simulink model "RealLifeTrainModel"  (R2024a)
settings: Solver=ode1  StartTime=0.0  StopTime=Inf  FixedStep=0.001  RelTol=1e-3
PostLoadFcn:
  | , if any(exist('dsrtsu_mdlpostloadfcn', 'file') ~= 0), dsrtsu_mdlpostloadfcn('Execute', bdroot); end,
InitFcn:
  | , if any(exist('rtifpga_mdlclblib', 'file') ~= 0), rtifpga_mdlclblib('Init', bdroot); end,
undefined symbols (not defined in the file): DiscIntNeverNeededParam
libraries: deeplib x29, svdutilitieslib x28, simulink x8, eeGeneralControl x8, rti1202lib_adc_class1 x6, rti1202serlib x5, spsEdgeDetectorLib x5, rtiemclib x2, rti1202lib_dac_class1 x1
(part 7 of 8)

== matlab function RealLifeTrainModel/ContractionMetricFilterSystem3/Normalize_Policy ==
  data: u input; y output
function y = fcn(u)

max_Fload =  569.629505294963
min_Fload = -610.339671010468

max_Fhyd = 729.261146885585
min_Fhyd = -777.489547410502

max_DFload = 123011.265014651
min_DFload = -142353.177843906

max_DFhyd = 219994.429294316
min_DFhyd = -270882.694509076

max_Pa = 12037835.3221229
min_Pa = 1849925.22965178

max_Pb = 14831789.6053956
min_Pb = 2808786.27887814

max_x = 0.082368752
min_x = 0.01990812

max_Dx = 0.682789396628826
min_Dx = -0.578996654196926

out = [1,1,1,1,1,1,1,1,1]

out(1) = (u(1) - min_Fhyd)/(max_Fhyd - min_Fhyd);
out(2) = (u(2) - min_DFhyd)/(max_DFhyd - min_DFhyd);
out(3) = (u(3) - min_Fload)/(max_Fload - min_Fload);
out(4) = (u(4) - min_DFload)/(max_DFload - min_DFload);
out(5) = (u(5) - min_Pa)/(max_Pa - min_Pa);
out(6) = (u(6) - min_Pb)/(max_Pb - min_Pb);
out(7) = (u(7) - min_x)/(max_x - min_x);
out(8) = (u(8) - min_Dx)/(max_Dx - min_Dx);

out(9) = (u(9) - min_Fload)/(max_Fload - min_Fload);


y = out;

== matlab function RealLifeTrainModel/ContractionMetricFilterSystem3/Policy_SS/Denormalize_Policy ==
  data: u input; y output
function y = fcn(u)

max_Fload =  569.629505294963
min_Fload = -610.339671010468

max_Fhyd = 729.261146885585
min_Fhyd = -777.489547410502

max_DFload = 123011.265014651
min_DFload = -142353.177843906

max_DFhyd = 219994.429294316
min_DFhyd = -270882.694509076

max_Pa = 12037835.3221229
min_Pa = 1849925.22965178

max_Pb = 14831789.6053956
min_Pb = 2808786.27887814

max_x = 0.082368752
min_x = 0.01990812

max_Dx = 0.682789396628826
min_Dx = -0.578996654196926

out = [1,1,1,1,1,1,1,1,1]

out(1) = (u(1))*(max_Fhyd - min_Fhyd) + min_Fhyd;

out(2) = (u(2))*(max_DFhyd - min_DFhyd) + min_DFhyd;

out(3) = (u(3))*(max_Fload - min_Fload) + min_Fload;

out(4) = (u(4))*(max_DFload - min_DFload) + min_DFload;

out(5) = (u(5))*(max_Pa - min_Pa) + min_Pa;

out(6) = (u(6))*(max_Pb - min_Pb) + min_Pb;

out(7) = (u(7))*(max_x - min_x) + min_x;

out(8) = (u(8))*(max_Dx - min_Dx) + min_Dx;

out(9) = (u(9))*(max_Fload - min_Fload) + min_Fload;


y = out;

== matlab function RealLifeTrainModel/ContractionMetricFilterSystem3/Policy_SS/FLcontroller1 ==
  data: pid input; y output; f input; g input; dFref input; d input; flag_start input
function y = fcn(pid,f,g,dFref,d,flag_start)

if flag_start == 1
    y = (dFref + pid - f)/g - d;
else 
    y = 1;
end

== matlab function RealLifeTrainModel/ContractionMetricFilterSystem3/Policy_SS/FunctionCalculateHydModel1 ==
  data: ixv input; f output; Pn input; Qn input; Un input; Vpl input; Ps input; Pt input; L_cyl input; Aa input; alfa input; c1 input; c2 input; Be input; flag_start input; data input; g output; force output
function [f,g,force] = fcn(ixv,Pn,Qn,Un,Vpl,Ps,Pt,L_cyl,Aa,alfa,c1,c2,Be,flag_start,data)
force = 0
if flag_start == 1
    Pa = data(5)
    Pb = data(6)
    xp = data(7)
    xpd = data(8)
    force = data(3)

    Kv = Qn/(Un*sqrt(Pn/2));
    
    Va = Vpl + Aa*xp;
    Vb = Vpl + (L_cyl - xp)*alfa*Aa;

    if(ixv >= 0)
        g = Be*Aa*Kv*( sign(Ps-Pa)*sqrt(abs(Ps-Pa))/Va + alfa*sign(Pb-Pt)*sqrt(abs(Pb-Pt))/Vb);
    else
        g = Be*Aa*Kv*( sign(Pa-Pt)*sqrt(abs(Pa-Pt))/Va + alfa*sign(Ps-Pb)*sqrt(abs(Ps-Pb))/Vb);
    end
    
    %g1 = Be*Aa*Kv*( sign(Ps-Pa)*sqrt(abs(Ps-Pa))/Va + alfa*sign(Pb-Pt)*sqrt(abs(Pb-Pt))/Vb);
    %g2 = Be*Aa*Kv*( sign(Pa-Pt)*sqrt(abs(Pa-Pt))/Va + alfa*sign(Ps-Pb)*sqrt(abs(Ps-Pb))/Vb);
    %g = (g1 + g2)/2;

    f = -Be*Aa^2*(((alfa)^2)/Vb + 1/Va)*xpd;
    
    g = c2*g;
    f = c1*f;
    
else
    f = 1;
    g = 1;
end

== matlab function RealLifeTrainModel/ContractionMetricFilterSystem3/Policy_SS/Policy ==
  data: u input; y output
function y = fcn(u)

y = (u)/2 + 0.5;

== matlab function RealLifeTrainModel/ContractionMetricFilterSystem3/Policy_SS/SmoothFnc1 ==
  data: u input; y output; smooth input
function y = fcn(u,smooth)
persistent last_value;

if(isempty(last_value))
    last_value = 0
end

y = smooth*last_value + (1 - smooth)*u
last_value = u

== matlab function RealLifeTrainModel/ContractionMetricFilterSystem3/Renormalize ==
  data: u input; y output
function y = fcn(u)

y = u*2 - 1;

== matlab function RealLifeTrainModel/MATLAB Function ==
  data: edge input; y output; last_value input; v output; last_value_counter input; last_value_recording input; x output; last_value_disturb input; last_value_z input; w output; e output
function [y,v,x,w,e] = fcn(edge,last_value,last_value_counter,last_value_recording,last_value_disturb,last_value_z)
y = 1;
if(edge == 1)
    y = 1;
    v = 0;
    x = 0;
    w = 0;
    e = 0;
else
    y = last_value;
    x = last_value_recording;
    v = last_value_counter;
    w = last_value_disturb;
    e = last_value_z;
end

== matlab function RealLifeTrainModel/MATLAB Sweep ==
  data: Time input; y output; Amp input; Freq input; StartTime input; EndTime input
function y = fcn(Time,Amp,Freq,StartTime,EndTime)
frequency = Freq/(2*(EndTime)) * (Time - StartTime);
y = Amp/2 - (Amp/2)*cos(2*3.1415*frequency*(Time - StartTime));

== matlab function RealLifeTrainModel/PolyDerivativeSubSystem1/MATLAB Function ==
  data: k input; dx output; Ts input; ddx output; dddx output; n_points input
function [dx,ddx,dddx] = poly_derivative(k,Ts,n_points)
    T =0 ;
    x = [k(1),k(2),k(3),k(4),k(5),k(6),k(7),k(8),k(9),k(10),k(11),k(12),k(13),k(14),k(15),k(16),k(17),k(18),k(19),k(20),k(21),k(22),k(23),k(24),k(25),k(26),k(27),k(28),k(29),k(30),k(31),k(32),k(33),k(34),k(35),k(36),k(37),k(38),k(39),k(40)];
    t = [T,T-1*Ts,T-2*Ts,T-3*Ts,T-4*Ts,T-5*Ts,T-6*Ts,T-7*Ts,T-8*Ts,T-9*Ts,T-10*Ts,T-11*Ts,T-12*Ts,T-13*Ts,T-14*Ts,T-15*Ts,T-16*Ts,T-17*Ts,T-18*Ts,T-19*Ts,T-20*Ts,T-21*Ts,T-22*Ts,T-23*Ts,T-24*Ts,T-25*Ts,T-26*Ts,T-27*Ts,T-28*Ts,T-29*Ts,T-30*Ts,T-31*Ts,T-32*Ts,T-33*Ts,T-34*Ts,T-35*Ts,T-36*Ts,T-37*Ts,T-38*Ts,T-39*Ts];

    p = polyfit(t(1:n_points), x(1:n_points), 3);    

    dp = polyder(p);         % derivative
    ddp = polyder(dp);
    dddp = polyder(ddp)
    
    dx = polyval(dp, T);     % evaluate at current time
    ddx = polyval(ddp, T)
    dddx = polyval(dddp, T)
end

== matlab function RealLifeTrainModel/PolyDerivativeSubSystem2/MATLAB Function ==
  data: k input; dx output; Ts input; ddx output; dddx output; n_points input
function [dx,ddx,dddx] = poly_derivative(k,Ts,n_points)
    T =0 ;
    x = [k(1),k(2),k(3),k(4),k(5),k(6),k(7),k(8),k(9),k(10),k(11),k(12),k(13),k(14),k(15),k(16),k(17),k(18),k(19),k(20),k(21),k(22),k(23),k(24),k(25),k(26),k(27),k(28),k(29),k(30),k(31),k(32),k(33),k(34),k(35),k(36),k(37),k(38),k(39),k(40)];
    t = [T,T-1*Ts,T-2*Ts,T-3*Ts,T-4*Ts,T-5*Ts,T-6*Ts,T-7*Ts,T-8*Ts,T-9*Ts,T-10*Ts,T-11*Ts,T-12*Ts,T-13*Ts,T-14*Ts,T-15*Ts,T-16*Ts,T-17*Ts,T-18*Ts,T-19*Ts,T-20*Ts,T-21*Ts,T-22*Ts,T-23*Ts,T-24*Ts,T-25*Ts,T-26*Ts,T-27*Ts,T-28*Ts,T-29*Ts,T-30*Ts,T-31*Ts,T-32*Ts,T-33*Ts,T-34*Ts,T-35*Ts,T-36*Ts,T-37*Ts,T-38*Ts,T-39*Ts];

    p = polyfit(t(1:n_points), x(1:n_points), 3);    

    dp = polyder(p);         % derivative
    ddp = polyder(dp);
    dddp = polyder(ddp)
    
    dx = polyval(dp, T);     % evaluate at current time
    ddx = polyval(ddp, T)
    dddx = polyval(dddp, T)
end

== matlab function RealLifeTrainModel/PolyDerivativeSubSystem3/MATLAB Function ==
  data: k input; dx output; Ts input; ddx output; dddx output; n_points input
function [dx,ddx,dddx] = poly_derivative(k,Ts,n_points)
    T =0 ;
    x = [k(1),k(2),k(3),k(4),k(5),k(6),k(7),k(8),k(9),k(10),k(11),k(12),k(13),k(14),k(15),k(16),k(17),k(18),k(19),k(20),k(21),k(22),k(23),k(24),k(25),k(26),k(27),k(28),k(29),k(30),k(31),k(32),k(33),k(34),k(35),k(36),k(37),k(38),k(39),k(40)];
    t = [T,T-1*Ts,T-2*Ts,T-3*Ts,T-4*Ts,T-5*Ts,T-6*Ts,T-7*Ts,T-8*Ts,T-9*Ts,T-10*Ts,T-11*Ts,T-12*Ts,T-13*Ts,T-14*Ts,T-15*Ts,T-16*Ts,T-17*Ts,T-18*Ts,T-19*Ts,T-20*Ts,T-21*Ts,T-22*Ts,T-23*Ts,T-24*Ts,T-25*Ts,T-26*Ts,T-27*Ts,T-28*Ts,T-29*Ts,T-30*Ts,T-31*Ts,T-32*Ts,T-33*Ts,T-34*Ts,T-35*Ts,T-36*Ts,T-37*Ts,T-38*Ts,T-39*Ts];

    p = polyfit(t(1:n_points), x(1:n_points), 3);    

    dp = polyder(p);         % derivative
    ddp = polyder(dp);
    dddp = polyder(ddp)
    
    dx = polyval(dp, T);     % evaluate at current time
    ddx = polyval(ddp, T)
    dddx = polyval(dddp, T)
end

== matlab function RealLifeTrainModel/CommSystem/SendMessageSystem/SendObs/CalcCrc ==
  data: u input; y output; length input
function y = fcn(u, length)
%#codegen

y = uint8(0);
length = length + 3;

for i = 1:length
    temp = (double(y) + double(u(i)))/2;  % safely add in double
    y = bitand(uint8(temp), uint8(255));  % clamp to 0-255, cast back to uint8
end

== matlab function RealLifeTrainModel/PolyDerivativeSubSystem5/MATLAB Function ==
  data: k input; dx output; Ts input; ddx output; dddx output; n_points input
function [dx,ddx,dddx] = poly_derivative(k,Ts,n_points)
    T =0 ;
    x = [k(1),k(2),k(3),k(4),k(5),k(6),k(7),k(8),k(9),k(10),k(11),k(12),k(13),k(14),k(15),k(16),k(17),k(18),k(19),k(20),k(21),k(22),k(23),k(24),k(25),k(26),k(27),k(28),k(29),k(30),k(31),k(32),k(33),k(34),k(35),k(36),k(37),k(38),k(39),k(40)];
    t = [T,T-1*Ts,T-2*Ts,T-3*Ts,T-4*Ts,T-5*Ts,T-6*Ts,T-7*Ts,T-8*Ts,T-9*Ts,T-10*Ts,T-11*Ts,T-12*Ts,T-13*Ts,T-14*Ts,T-15*Ts,T-16*Ts,T-17*Ts,T-18*Ts,T-19*Ts,T-20*Ts,T-21*Ts,T-22*Ts,T-23*Ts,T-24*Ts,T-25*Ts,T-26*Ts,T-27*Ts,T-28*Ts,T-29*Ts,T-30*Ts,T-31*Ts,T-32*Ts,T-33*Ts,T-34*Ts,T-35*Ts,T-36*Ts,T-37*Ts,T-38*Ts,T-39*Ts];

    p = polyfit(t(1:n_points), x(1:n_points), 3);    

    dp = polyder(p);         % derivative
    ddp = polyder(dp);
    dddp = polyder(ddp)
    
    dx = polyval(dp, T);     % evaluate at current time
    ddx = polyval(ddp, T)
    dddx = polyval(dddp, T)
end

== matlab function RealLifeTrainModel/PolyDerivativeSubSystem6/MATLAB Function ==
  data: k input; dx output; Ts input; ddx output; dddx output
function [dx,ddx,dddx] = poly_derivative(k,Ts)
    T =0 ;
    x = [k(1),k(2),k(3),k(4),k(5),k(6),k(7),k(8),k(9),k(10),k(11),k(12),k(13),k(14),k(15),k(16),k(17),k(18),k(19),k(20)];
    t = [T,T-1*Ts,T-2*Ts,T-3*Ts,T-4*Ts,T-5*Ts,T-6*Ts,T-7*Ts,T-8*Ts,T-9*Ts,T-10*Ts,T-11*Ts,T-12*Ts,T-13*Ts,T-14*Ts,T-15*Ts,T-16*Ts,T-17*Ts,T-18*Ts,T-19*Ts];

    p = polyfit(t, x, 3);    

    dp = polyder(p);         % derivative
    ddp = polyder(dp);
    dddp = polyder(ddp)
    
    dx = polyval(dp, T);     % evaluate at current time
    ddx = polyval(ddp, T)
    dddx = polyval(dddp, T)
end

== matlab function RealLifeTrainModel/MATLAB Function4 ==
  data: u1 input; y output; u2 input; new_u1 output; u3 input; u4 input
function [y, new_u1] = fcn(u1, u2,u3,u4)
% u1: current counter (from Data Store Read)
% u2: threshold (e.g. 10)
% y: enable signal
% new_u1: updated counter value (for Data Store Write)
if(u4)
    u1=0
end

new_u1 = u1

y = 0
if(u3)
    if u1 >= u2
        y = 1;
        new_u1 = 0;
    else
        y = 0;
        new_u1 = u1 + 1;
    end
end

== matlab function RealLifeTrainModel/FLcontroller1 ==
  data: pid input; y output; f input; g input; dFref input; d input; flag_start input
function y = fcn(pid,f,g,dFref,d,flag_start)

if flag_start == 1
    y = (dFref + pid - f)/g - d;
else 
    y = 1;
end

== matlab function RealLifeTrainModel/Interrupt-Driven Reception/ScaleData ==
  data: u input; y output; max input; min input
function y = fcn(u,max,min)

y = u*(max - min) + min;

== matlab function RealLifeTrainModel/ContractionMetricFilterSystem2/MATLAB Function ==
  data: x input; u_filtered output; ref input; u_nom input; dt input; task_dim input; row_major input; td_is_zero_based input; eps_pd input; use_A_transpose input; lambda_val input; last_ixv input; flag_start input; Kp input; Ki input; ref_denorm input; Dref_denorm input; integral_erro input; cert_val output; is_active output; a_val output; b_val output; du_out output; M_curr_out output; Mdot_out output; erro output; u_nom_teste output; A_m output; B_m output; K_m output; k1 input; k2 input; k3 input
function [u_filtered, cert_val, is_active, a_val, b_val, du_out, M_curr_out, Mdot_out,erro,u_nom_teste,A_m,B_m,K_m] = ...
    qp_filter_projected_deltaU_getM( ...
        x, ref, u_nom, ...
        dt, task_dim, ...
        row_major, td_is_zero_based, eps_pd, use_A_transpose, lambda_val, ...
        last_ixv, flag_start, Kp, Ki, ref_denorm, Dref_denorm,integral_erro,k1,k2,k3) %#codegen

max_Fload =  569.629505294963
min_Fload = -610.339671010468

% Closed-form QP:  min 0.5*||Δu||^2  s.t. a'*Δu <= b,   u_filt = u_nom + Δu
% Uses your get_M(x) to build M(x) internally (no M_* inputs).
% A,B from FD on get_model([x;u]), K from FD on your policy(...).

% -------- defaults / casts (codegen-safe) --------
if nargin < 6  || isempty(row_major),        row_major        = true;  end %#ok<NASGU> % kept for API compat; get_M already fixes orientation
if nargin < 7  || isempty(td_is_zero_based), td_is_zero_based = true;  end
if nargin < 8  || isempty(eps_pd),           eps_pd           = single(1e-3); end
if nargin < 9  || isempty(use_A_transpose),  use_A_transpose  = false; end

tdZeroBased = (td_is_zero_based ~= 0);
useAT       = (use_A_transpose  ~= 0);

dt          = cast(dt,          'single');
eps_pd      = cast(eps_pd,      'single');
lambda_val  = cast(lambda_val,  'single');
Kp          = cast(Kp,          'single');
Ki          = cast(Ki,          'single');
ref_denorm  = cast(ref_denorm,  'single');
Dref_denorm = cast(Dref_denorm, 'single');
last_ixv    = cast(last_ixv,    'single');
flag_start  = cast(flag_start,  'single');

% -------- sizes / shapes --------
n   = int32(8);                 % state dim
m   = int32(1);                 % scalar control
x_m = reshape(x, [], 1);        % (n x 1), normalized [0,1]

% -------- Metric from your network --------
M_curr = cast(get_M(x_m), 'single');    % (8x8) SPD already
M_curr_out = M_curr;                    % expose for debug

% -------- Compute Mdot --------
persistent have_prev M_prev
if isempty(have_prev)
    have_prev = false;
    M_prev    = zeros(8,8,'single');
end

if flag_start ~= 0
    % reset at episode start
    have_prev = false;
end


M_dot = (M_curr - M_prev) ./ dt;    % time FD


% update persistent for next call
M_prev    = M_curr;
have_prev = true;

Mdot_out = M_dot;    % expose for debug

%policy(normdata,last_ixv,flag_start,ref_denorm,Kp,Ki,Dref_denorm,integral)
u_nom_teste = 2*policy_nominal_(x_m,ref,last_ixv,flag_start,Kp,Ki,ref_denorm,Dref_denorm,integral_erro) - 1

% -------- Linearize model: A = ∂f/∂x, B = ∂f/∂u --------
[A_m, B_m] = linearize_model_fd_(x_m, u_nom, n);

% -------- K from your policy (FD) --------

K_m = policy_jacobian_fd_(x_m, ref, last_ixv, flag_start, Kp, Ki, ref_denorm, Dref_denorm, n,integral_erro); % (1 x n)

% -------- ABK (+ optional Aᵀ) --------
A_use = A_m; if useAT, A_use = A_m.'; end
ABK   = A_use + B_m * K_m;     % (n x n)

% -------- Contraction matrix --------
symPart = M_curr * ABK;
symPart = symPart + symPart.'; 
C = M_dot + symPart + (2 * lambda_val) * M_curr;

% -------- contracting direction v --------
td = int32(task_dim); if tdZeroBased, td = td + 1; end
td = max(1, min(td, n));
v = zeros(n,1,'single');
v(td,1) = cast(x_m(td,1) - cast(ref,'like',x_m), 'single');

% -------- certificate & halfspace --------
cert_val = cast(v' * C * v, 'like', u_nom);      % scalar
a_row    = 2 * (v' * (M_curr * B_m));            % (1 x m)
e = ref - x(3)
b_val    = cast(-(v' * C * v), 'like', u_nom) - (k2 + k3*abs(e));   % scalar

% -------- closed-form projection in Δu-space --------
a_col  = cast(a_row.', 'like', u_nom);           % (m x 1)
anorm2 = max(cast(1e-12, 'like', u_nom), sum(a_col .* a_col));

if b_val >= 0
    du = zeros(m, 1, 'like', u_nom); active = 0;
else
    du = (b_val / anorm2) * a_col;   active = 1;
end

% elementwise clip Δu
du = min(max(du, -eps_pd), eps_pd);

u_filtered = u_nom + du + k1*(e);
is_active  = double(active);
a_val      = a_col;
du_out     = du;

force = x(3)*(max_Fload - min_Fload) + min_Fload

erro = ref_denorm - force
end

% ====================== helpers (codegen-safe) ======================

function y = clip01_(z)
% clamp to [0,1] (single, vector/scalar)
y = min(max(cast(z,'single'), cast(0,'single')), cast(1,'single'));
end

function [A_m, B_m] = linearize_model_fd_(x, u, n)
% Central FD on your ONNX-backed model get_model([x;u])
x = cast(x, 'single'); u = cast(u, 'single');
A_m = zeros(n, n, 'single');
B_m = zeros(n, 1, 'single');

eps_x = cast(1e-4, 'single');
eps_u = cast(1e-3, 'single');

xm = clip01_(x);
f = f_model_(x, u);

% A: ∂f/∂x
for i = 1:n
    dx = zeros(n,1,'single'); dx(i) = eps_x;
    xp = (x + dx);

    fp = f_model_(xp, u);

    A_m(:, i) = (fp - f) ./ (eps_x);
end

% B: ∂f/∂u
up = (u + eps_u);
ul = (u - eps_u);
xm = clip01_(x);
fp = f_model_(x, up);
fl = f_model_(x, ul);

B_m(:, 1) = (fp - f) ./ (eps_u);
end

function f = f_model_(x, u)
% Evaluate learned dynamics at (x,u); get_model expects 9x1 input [x; u]
xu = [cast(x,'single'); cast(u,'single')];
f  = cast(get_model(xu), 'single');   % (8x1)
end

function K = policy_jacobian_fd_(x, ref, last_ixv, flag_start, Kp, Ki, ref_denorm, Dref_denorm, n,integral)
% Central FD of your policy π(x, ref) using your provided function
K = zeros(1, n, 'single');
eps_x = cast(1e-3, 'single');
x_ = (x);
u = policy_nominal_(x_, ref, last_ixv, flag_start, Kp, Ki, ref_denorm, Dref_denorm,integral);

for i = 1:n
    dx = zeros(n,1,'single'); dx(i) = eps_x;
    xp = (x + dx);

    up = policy_nominal_(xp, ref, last_ixv, flag_start, Kp, Ki, ref_denorm, Dref_denorm,integral);

    K(1,i) = (up - u) ./ (eps_x);
end
end

function u = policy_nominal_(x, ref, last_ixv, flag_start, Kp, Ki, ref_denorm, Dref_denorm,integral)
% Thin wrapper to your policy(normdata,last_ixv,flag_start,ref_denorm,Kp,Ki,Dref_denorm)
normdata = [cast(x,'single'); cast(ref,'single')];  % 9x1, normalized
u = cast(policy(normdata, last_ixv, flag_start, ref_denorm, Kp, Ki, Dref_denorm,integral), 'single');
end


function y = get_model(x)
%#codegen
% x: 9x1 normalized in [0,1]
% y: 8x1 single, normalized to [0,1]
% y = y1 + (y2.^2) * u_scalar, then re-scale to [0,1]

% ---- normalize / split inputs ----
x_single = single(x(:));           % 9x1
x_scaled = 2*x_single - 1;         % [-1, 1]
feat     = x_scaled(1:8);          % 8x1
u_scalar = x_scaled(9);            % scalar

% ---- two pure-C forwards using saved weights ----
y1 = model_forward_m1(feat);       % 8x1
y2 = model_forward_m2(feat);       % 8x1

% ---- combine and clamp ----
y  = y1 + (y2 .* y2) * u_scalar;   % 8x1
y  = 0.5 * y + 0.5;                % back to [0,1]
end


function M = get_M(x)
%#codegen
% x: 8x1 normalized in [0,1]
% M: 8x8 SPD single

x8  = single(x(:));                % 8x1

% metric net: 2-FC (64 outputs) → reshape to 8x8
v64 = metric_forward_2fc(x8);      % 64x1

n    = int32(8);
Mraw = reshape(v64, [n, n]).';                          % row-major → col-major
M    = (Mraw.' * Mraw) + single(1e-3) * eye(n,'single'); % SPD
end


% ==================== helpers (pure C, RTI-safe) ====================

function y = model_forward_m1(x8)
%#codegen
% 3-FC with ReLU after first two; outputs 8x1
persistent W1 b1 W2 b2 W3 b3 init
if isempty(init)
    S  = coder.load(coder.const('C:\Users\ic2d\Documents\GitHub\dSpace_Controllers_legged\model_1_weights.mat'));
    W1 = single(S.W1);  b1 = single(S.b1);   % [64x8],  [64x1]
    W2 = single(S.W2);  b2 = single(S.b2);   % [64x64], [64x1]
    W3 = single(S.W3);  b3 = single(S.b3);   % [8x64],  [8x1]
    init = true;
end
x8 = single(x8(:));
z1 = W1 * x8 + b1;   a1 = max(z1, single(0));   % ReLU
z2 = W2 * a1 + b2;   a2 = max(z2, single(0));   % ReLU
y  = W3 * a2 + b3;                              % 8x1
end

function y = model_forward_m2(x8)
%#codegen
% 3-FC with ReLU after first two; outputs 8x1
persistent W1 b1 W2 b2 W3 b3 init
if isempty(init)
    S  = coder.load(coder.const('C:\Users\ic2d\Documents\GitHub\dSpace_Controllers_legged\model_2_weights.mat'));
    W1 = single(S.W1);  b1 = single(S.b1);   % [64x8],  [64x1]
    W2 = single(S.W2);  b2 = single(S.b2);   % [64x64], [64x1]
    W3 = single(S.W3);  b3 = single(S.b3);   % [8x64],  [8x1]
    init = true;
end
x8 = single(x8(:));
z1 = W1 * x8 + b1;   a1 = max(z1, single(0));   % ReLU
z2 = W2 * a1 + b2;   a2 = max(z2, single(0));   % ReLU
y  = W3 * a2 + b3;                              % 8x1
end

function y64 = metric_forward_2fc(x8)
%#codegen
% 2-FC with ReLU after first; outputs 64x1
persistent W1 b1 W2 b2 init
if isempty(init)
    S  = coder.load(coder.const('C:\Users\ic2d\Documents\GitHub\dSpace_Controllers_legged\metric_weights.mat'));
    W1 = single(S.W1);  b1 = single(S.b1);   % [64x8],  [64x1]
    W2 = single(S.W2);  b2 = single(S.b2);   % [64x64], [64x1]
    init = true;
end
x8  = single(x8(:));
z1  = W1 * x8 + b1;                 % [64x1]
a1  = max(z1, single(0));           % ReLU
y64 = W2 * a1 + b2;                 % [64x1]
end


function y = policy(normdata,last_ixv,flag_start,ref_denorm,Kp,Ki,Dref_denorm,integral)

data = denorm(normdata)

y = FL(last_ixv,flag_start,data, Kp,Ki,Dref_denorm,ref_denorm,integral);

end


function y = denorm(u)
    max_Fload =  569.629505294963
    min_Fload = -610.339671010468
    
    max_Fhyd = 729.261146885585
    min_Fhyd = -777.489547410502
    
    max_DFload = 123011.265014651
    min_DFload = -142353.177843906
    
    max_DFhyd = 219994.429294316
    min_DFhyd = -270882.694509076
    
    max_Pa = 12037835.3221229
    min_Pa = 1849925.22965178
    
    max_Pb = 14831789.6053956
    min_Pb = 2808786.27887814
    
    max_x = 0.082368752
    min_x = 0.01990812
    
    max_Dx = 0.682789396628826
    min_Dx = -0.578996654196926
    
    out = [1,1,1,1,1,1,1,1,1]
    
    out(1) = (u(1))*(max_Fhyd - min_Fhyd) + min_Fhyd;
    
    out(2) = (u(2))*(max_DFhyd - min_DFhyd) + min_DFhyd;
    
    out(3) = (u(3))*(max_Fload - min_Fload) + min_Fload;
    
    out(4) = (u(4))*(max_DFload - min_DFload) + min_DFload;
    
    out(5) = (u(5))*(max_Pa - min_Pa) + min_Pa;
    
    out(6) = (u(6))*(max_Pb - min_Pb) + min_Pb;
    
    out(7) = (u(7))*(max_x - min_x) + min_x;
    
    out(8) = (u(8))*(max_Dx - min_Dx) + min_Dx;
    
    out(9) = (u(9))*(max_Fload - min_Fload) + min_Fload;
    
    
    y = out;
end

function y = FL(ixv,flag_start,data_denorm,Kp,Ki,Dref_denorm,Ref_denorm,integral)
    Pn = 7000000
    Qn = 10/60000
    Un = 0.05
    Be = 1.31E+9
    c1 = 1
    c2 = 1
    alfa = 0.609
    Vpl = 0.00121
    Ps = 16000000
    Pt = 0
    L_cyl = 0.08
    Aa = 0.000201
    
    if flag_start == 1
        data = data_denorm
        Pa = data(5)
        Pb = data(6)
        xp = data(7)
        xpd = data(8)
    
        Kv = Qn/(Un*sqrt(Pn/2));
        
        Va = Vpl + Aa*xp;
        Vb = Vpl + (L_cyl - xp)*alfa*Aa;
    
        if(ixv >= 0)
            g = Be*Aa*Kv*( sign(Ps-Pa)*sqrt(abs(Ps-Pa))/Va + alfa*sign(Pb-Pt)*sqrt(abs(Pb-Pt))/Vb);
        else
            g = Be*Aa*Kv*( sign(Pa-Pt)*sqrt(abs(Pa-Pt))/Va + alfa*sign(Ps-Pb)*sqrt(abs(Ps-Pb))/Vb);
        end
        
        %g1 = Be*Aa*Kv*( sign(Ps-Pa)*sqrt(abs(Ps-Pa))/Va + alfa*sign(Pb-Pt)*sqrt(abs(Pb-Pt))/Vb);
        %g2 = Be*Aa*Kv*( sign(Pa-Pt)*sqrt(abs(Pa-Pt))/Va + alfa*sign(Ps-Pb)*sqrt(abs(Ps-Pb))/Vb);
        %g = (g1 + g2)/2;
    
        f = -Be*Aa^2*(((alfa)^2)/Vb + 1/Va)*xpd;
        
        g = c2*g;
        f = c1*f;
    
    
        y = (-c1*f + Dref_denorm + Kp*(Ref_denorm - data(3)) + Ki*integral)/(c2*g)
        y = y/0.05;
        y = y/2 + 0.5

    else
        y = single(0)
    end
end

== matlab function RealLifeTrainModel/RefRand ==
  data: flag input; new_amp output; amp input; freq input; new_freq output; random input; max_freq input; pos input; new_pos output; start_freq input
function [new_amp,new_freq,new_pos] = fcn(flag,amp,freq,random,max_freq,pos,start_freq)

new_amp = amp;
new_freq = freq;
new_pos = pos;

if flag == 1
    % Define min and max for each parameter

    pos_min = -50; 
    pos_max = -50 + random * 50;

    % Create 6 discrete values
    amp_values  = [200,300,400];
    freq_values = [0.5, 1 ,1.5 ,2 ,2.5 ,3];

    amp_values  = [start_freq,start_freq,start_freq];
    freq_values = [max_freq, max_freq ,max_freq ,max_freq ,max_freq ,max_freq];

    pos_values  = linspace(pos_min, pos_max, 6);

    % Randomly pick one of the 6
    new_amp  = amp_values(randi(3));
    new_freq = freq_values(randi(6));
    new_pos  = pos_values(randi(6));
end

== matlab function RealLifeTrainModel/Interrupt-Driven Reception/ScaleData1 ==
  data: u input; y output; max input; min input
function y = fcn(u,max,min)

y = u*(max - min) + min;

== matlab function RealLifeTrainModel/RL_FL ==
  data: g input; erro input; y output; Kp input; Ki input; int_erro input; flag_start input
function y = fcn(g,erro,Kp,Ki,int_erro,flag_start)

if flag_start == 1
    y = (Kp*erro + Ki*int_erro)/g;
else 
    y = 1;
end

== matlab function RealLifeTrainModel/ContractionMetricFilterSystem2/NormalizeMetric_1 ==
  data: u input; y output
function y = fcn(u)

max_Fload =  569.629505294963
min_Fload = -610.339671010468

max_Fhyd = 729.261146885585
min_Fhyd = -777.489547410502

max_DFload = 123011.265014651
min_DFload = -142353.177843906

max_DFhyd = 219994.429294316
min_DFhyd = -270882.694509076

max_Pa = 12037835.3221229
min_Pa = 1849925.22965178

max_Pb = 14831789.6053956
min_Pb = 2808786.27887814

max_x = 0.082368752
min_x = 0.01990812

max_Dx = 0.682789396628826
min_Dx = -0.578996654196926

out = [1,1,1,1,1,1,1,1]

out(1) = (u(1) - min_Fhyd)/(max_Fhyd - min_Fhyd);
out(2) = (u(2) - min_DFhyd)/(max_DFhyd - min_DFhyd);
out(3) = (u(3) - min_Fload)/(max_Fload - min_Fload);
out(4) = (u(4) - min_DFload)/(max_DFload - min_DFload);
out(5) = (u(5) - min_Pa)/(max_Pa - min_Pa);
out(6) = (u(6) - min_Pb)/(max_Pb - min_Pb);
out(7) = (u(7) - min_x)/(max_x - min_x);
out(8) = (u(8) - min_Dx)/(max_Dx - min_Dx);



y = out;

== matlab function RealLifeTrainModel/ContractionMetricFilterSystem2/NormalizeMetric_2 ==
  data: u input; y output
function y = fcn(u)

max_Fload =  569.629505294963
min_Fload = -610.339671010468

max_Fhyd = 729.261146885585
min_Fhyd = -777.489547410502

max_DFload = 123011.265014651
min_DFload = -142353.177843906

max_DFhyd = 219994.429294316
min_DFhyd = -270882.694509076

max_Pa = 12037835.3221229
min_Pa = 1849925.22965178

max_Pb = 14831789.6053956
min_Pb = 2808786.27887814

max_x = 0.082368752
min_x = 0.01990812

max_Dx = 0.682789396628826
min_Dx = -0.578996654196926

out = [1]


out(1) = (u(1) - min_Fload)/(max_Fload - min_Fload);




y = out;

== matlab function RealLifeTrainModel/ContractionMetricFilterSystem2/Normalize_Policy ==
  data: u input; y output
function y = fcn(u)

max_Fload =  569.629505294963
min_Fload = -610.339671010468

max_Fhyd = 729.261146885585
min_Fhyd = -777.489547410502

max_DFload = 123011.265014651
min_DFload = -142353.177843906

max_DFhyd = 219994.429294316
min_DFhyd = -270882.694509076

max_Pa = 12037835.3221229
min_Pa = 1849925.22965178

max_Pb = 14831789.6053956
min_Pb = 2808786.27887814

max_x = 0.082368752
min_x = 0.01990812

max_Dx = 0.682789396628826
min_Dx = -0.578996654196926

out = [1,1,1,1,1,1,1,1,1]

out(1) = (u(1) - min_Fhyd)/(max_Fhyd - min_Fhyd);
out(2) = (u(2) - min_DFhyd)/(max_DFhyd - min_DFhyd);
out(3) = (u(3) - min_Fload)/(max_Fload - min_Fload);
out(4) = (u(4) - min_DFload)/(max_DFload - min_DFload);
out(5) = (u(5) - min_Pa)/(max_Pa - min_Pa);
out(6) = (u(6) - min_Pb)/(max_Pb - min_Pb);
out(7) = (u(7) - min_x)/(max_x - min_x);
out(8) = (u(8) - min_Dx)/(max_Dx - min_Dx);

out(9) = (u(9) - min_Fload)/(max_Fload - min_Fload);


y = out;

== matlab function RealLifeTrainModel/Interrupt-Driven Reception/ProcessCmd ==
  data: flag_receive input; y output; cmd input; flag_start input uint8; flag_abort input uint8; new_flag_start output uint8; new_flag_abort output uint8; flag_start_train input uint8; new_flag_start_train output uint8; new_flag_ack output uint8; flag_ack input uint8
function [y,new_flag_start,new_flag_abort,new_flag_start_train,new_flag_ack] = fcn(flag_receive,cmd,flag_start,flag_abort,flag_start_train,flag_ack)

y = 0;

new_flag_start = flag_start;
new_flag_abort = flag_abort;
new_flag_start_train = flag_start_train;
new_flag_ack = flag_ack;


CMD_RECEIVING_DATA_OBS = 0x01;
CMD_ABORT_EPISODE = 0x02;
CMD_START_EPISODE = 0x03;
CMD_STOP_EPISODE = 0x04;
CMD_START_TRAINING = 0x05;
CMD_STOP_TRAINING = 0x06;
CMD_ACKNOWLEDGE = 0x07;

if(flag_receive)
    if(cmd == CMD_START_EPISODE)
        new_flag_start = uint8(1);
        new_flag_abort = uint8(0);
        new_flag_ack = uint8(1);
    end

    if(cmd == CMD_START_TRAINING)
        new_flag_start_train = uint8(1);
        new_flag_start = uint8(1);
        new_flag_abort = uint8(0);
        new_flag_ack = uint8(1);
    end

    if(cmd == CMD_STOP_EPISODE)
        new_flag_start = uint8(0);
        new_flag_ack = uint8(1);
    end

    if(cmd == CMD_STOP_TRAINING)
        new_flag_start_train = uint8(0);
        new_flag_start = uint8(0);
        new_flag_abort = uint8(1);
        new_flag_ack = uint8(1);
    end

    if(cmd == CMD_ACKNOWLEDGE)
        new_flag_ack = uint8(1);
    end


    y = 1;
end

== matlab function RealLifeTrainModel/Interrupt-Driven Reception/SerialReceiveStateMachine ==
  data: data input; mss_received output; length input; crc input; step input; new_step output; new_crc output; new_length output; cmd input; new_cmd output; length_data input; new_length_data output; new_data_rcv output; data_rcv input; data_rcv2 input; new_data_rcv2 output
function [mss_received,new_step,new_crc,new_length,new_cmd,new_length_data,new_data_rcv,new_data_rcv2] = fcn(data,length,crc,step,cmd,length_data,data_rcv,data_rcv2)

START_BYTE = 0xD4;
END_BYTE = 0xB1;
mss_received = uint8(0);

CMD_RECEIVING_DATA_OBS = 0x01;
CMD_ABORT_EPISODE = 0x02;
CMD_START_EPISODE = 0x03;
CMD_STOP_EPISODE = 0x04;
CMD_START_TRAINING = 0x05;
CMD_STOP_TRAINING = 0x06;
CMD_ACKNOWLEDGE = 0x07;

StartByteStep = 0;
LengthStep = 1;
CmdStep = 2;
DataStep = 3;
CrcStep = 4;
EndByteStep = 5;

counter = 0;

new_data_rcv = data_rcv;
new_data_rcv2 = data_rcv2;

step = cast(0,"uint8");

for i = 1:length
    switch step
        case StartByteStep
            if(data(i) == START_BYTE)
                mss_received = cast(0,"uint8");
                step = cast(LengthStep,"uint8");
                crc = cast(0,"uint8");
                length = cast(0,"uint8");
                crc = bitand((crc + data(i))/2, 255);
            end
        
        case LengthStep
            length_data = cast(data(i),"uint8");
            crc = bitand((crc + data(i))/2, 255);
            step = cast(CmdStep,"uint8");

        case CmdStep
            cmd = cast(data(i),"uint8");
            crc = bitand((crc + data(i))/2, 255);
            if(length_data == 0)
                step = cast(CrcStep,"uint8");
            else
                step = cast(DataStep,"uint8");
            end
        case DataStep
            if(counter == (length_data - 1))
                if(cmd == 7)
                    new_data_rcv2 = cast(data(i),"uint8");
                    step = cast(CrcStep,"uint8");
                else 
                    new_data_rcv2 = data_rcv2;
                    step = cast(CrcStep,"uint8");
                end
            else
                if(cmd == 7)
                    new_data_rcv = cast(data(i),"uint8");
                    counter = counter + 1;
                else
                    new_data_rcv = data_rcv;
                    counter = counter + 1;
                end
            end
            crc = bitand((crc + data(i))/2, 255);

        case CrcStep
            if(data(i) == (crc))
                step = cast(EndByteStep,"uint8");
            else
                %cmd = cast(0,"uint8");
                crc = cast(0,"uint8");
                step = cast(EndByteStep,"uint8");
            end
        

        case EndByteStep
            if(data(i) == END_BYTE)
                mss_received = cast(1,"uint8");
                %crc = cast(0,"uint8");
                step = cast(StartByteStep,"uint8");
            else
                %crc = cast(0,"uint8");
                cmd = cast(0,"uint8");
                step = cast(StartByteStep,"uint8");
            end

       
            
    end
    

end

new_length_data = length_data;
new_step = step;
new_crc = crc;
new_length = length;
new_cmd = cmd;

== matlab function RealLifeTrainModel/CommSystem/SendMessageSystem/CancelSubsystem/MATLAB Function ==
  data: counter input; cancel output; limit input; new_counter output
function [cancel,new_counter] = fcn(counter,limit)
new_counter = counter;
cancel = 0

if(counter >= limit)
cancel = 1
else
new_counter = counter + 1
end

== matlab function RealLifeTrainModel/RefFunctionSin ==
  data: Time input; y output; Amp input; Freq input; StartTime input; EndTime input; new_amp output
function [y,new_amp] = fcn(Time,Amp,Freq,StartTime,EndTime)

new_amp = Amp
rep = fix(14*Freq)

rest = rem(rep, Freq)

time_var = rep/Freq

if((Time - StartTime) < 4)
    y = 0;
elseif ((Time - StartTime) > (4 + time_var))
    new_amp = 0
    y = 0;
else 
    y = (Amp/2) - (Amp/2)*cos(2*3.1415*Freq*(Time - 4 - StartTime));
end

== matlab function RealLifeTrainModel/ContractionMetricFilterSystem2/Policy_SS/Denormalize_Policy ==
  data: u input; y output
function y = fcn(u)

max_Fload =  569.629505294963
min_Fload = -610.339671010468

max_Fhyd = 729.261146885585
min_Fhyd = -777.489547410502

max_DFload = 123011.265014651
min_DFload = -142353.177843906

max_DFhyd = 219994.429294316
min_DFhyd = -270882.694509076

max_Pa = 12037835.3221229
min_Pa = 1849925.22965178

max_Pb = 14831789.6053956
min_Pb = 2808786.27887814

max_x = 0.082368752
min_x = 0.01990812

max_Dx = 0.682789396628826
min_Dx = -0.578996654196926

out = [1,1,1,1,1,1,1,1,1]

out(1) = (u(1))*(max_Fhyd - min_Fhyd) + min_Fhyd;

out(2) = (u(2))*(max_DFhyd - min_DFhyd) + min_DFhyd;

out(3) = (u(3))*(max_Fload - min_Fload) + min_Fload;

out(4) = (u(4))*(max_DFload - min_DFload) + min_DFload;

out(5) = (u(5))*(max_Pa - min_Pa) + min_Pa;

out(6) = (u(6))*(max_Pb - min_Pb) + min_Pb;

out(7) = (u(7))*(max_x - min_x) + min_x;

out(8) = (u(8))*(max_Dx - min_Dx) + min_Dx;

out(9) = (u(9))*(max_Fload - min_Fload) + min_Fload;


y = out;

== matlab function RealLifeTrainModel/ContractionMetricFilterSystem2/Policy_SS/FLcontroller1 ==
  data: pid input; y output; f input; g input; dFref input; d input; flag_start input
function y = fcn(pid,f,g,dFref,d,flag_start)

if flag_start == 1
    y = (dFref + pid - f)/g - d;
else 
    y = 1;
end

== matlab function RealLifeTrainModel/ContractionMetricFilterSystem2/Policy_SS/FunctionCalculateHydModel1 ==
  data: ixv input; f output; Pn input; Qn input; Un input; Vpl input; Ps input; Pt input; L_cyl input; Aa input; alfa input; c1 input; c2 input; Be input; flag_start input; data input; g output; force output
function [f,g,force] = fcn(ixv,Pn,Qn,Un,Vpl,Ps,Pt,L_cyl,Aa,alfa,c1,c2,Be,flag_start,data)
force = 0
if flag_start == 1
    Pa = data(5)
    Pb = data(6)
    xp = data(7)
    xpd = data(8)
    force = data(3)

    Kv = Qn/(Un*sqrt(Pn/2));
    
    Va = Vpl + Aa*xp;
    Vb = Vpl + (L_cyl - xp)*alfa*Aa;

    if(ixv >= 0)
        g = Be*Aa*Kv*( sign(Ps-Pa)*sqrt(abs(Ps-Pa))/Va + alfa*sign(Pb-Pt)*sqrt(abs(Pb-Pt))/Vb);
    else
        g = Be*Aa*Kv*( sign(Pa-Pt)*sqrt(abs(Pa-Pt))/Va + alfa*sign(Ps-Pb)*sqrt(abs(Ps-Pb))/Vb);
    end
    
    %g1 = Be*Aa*Kv*( sign(Ps-Pa)*sqrt(abs(Ps-Pa))/Va + alfa*sign(Pb-Pt)*sqrt(abs(Pb-Pt))/Vb);
    %g2 = Be*Aa*Kv*( sign(Pa-Pt)*sqrt(abs(Pa-Pt))/Va + alfa*sign(Ps-Pb)*sqrt(abs(Ps-Pb))/Vb);
    %g = (g1 + g2)/2;

    f = -Be*Aa^2*(((alfa)^2)/Vb + 1/Va)*xpd;
    
    g = c2*g;
    f = c1*f;
    
else
    f = 1;
    g = 1;
end

== matlab function RealLifeTrainModel/ContractionMetricFilterSystem2/Policy_SS/Policy ==
  data: u input; y output
function y = fcn(u)

y = (u)/2 + 0.5;

== matlab function RealLifeTrainModel/CommSystem/SendMessageSystem/SendObs/Norm ==
  data: u input; y output; max input; min input
function y = fcn(u,max,min)

y = (u - min)/(max - min);

== matlab function RealLifeTrainModel/CommSystem/SendMessageSystem/SendObs/Norm1 ==
  data: u input; y output; max input; min input
function y = fcn(u,max,min)

y = (u - min)/(max - min);

== matlab function RealLifeTrainModel/CommSystem/SendMessageSystem/SendObs/Norm10 ==
  data: u input; y output; max input; min input
function y = fcn(u,max,min)

y = (u - min)/(max - min);

== matlab function RealLifeTrainModel/CommSystem/SendMessageSystem/SendObs/Norm11 ==
  data: u input; y output; max input; min input
function y = fcn(u,max,min)

y = (u - min)/(max - min);

== matlab function RealLifeTrainModel/CommSystem/SendMessageSystem/SendObs/Norm2 ==
  data: u input; y output; max input; min input
function y = fcn(u,max,min)

y = (u - min)/(max - min);

== matlab function RealLifeTrainModel/CommSystem/SendMessageSystem/SendObs/Norm3 ==
  data: u input; y output; max input; min input
function y = fcn(u,max,min)

y = (u - min)/(max - min);

== matlab function RealLifeTrainModel/CommSystem/SendMessageSystem/SendObs/Norm4 ==
  data: u input; y output; max input; min input
function y = fcn(u,max,min)

y = (u - min)/(max - min);

== matlab function RealLifeTrainModel/CommSystem/SendMessageSystem/SendObs/Norm5 ==
  data: u input; y output; max input; min input
function y = fcn(u,max,min)

y = (u - min)/(max - min);

== matlab function RealLifeTrainModel/SetStartTime ==
  data: flag input; start_time output; time input; start input
function start_time = fcn(flag,time,start)

if(flag == 1)
    start_time = time;
else
    start_time = start;
end

== matlab function RealLifeTrainModel/CommSystem/SendMessageSystem/SendObs/Norm6 ==
  data: u input; y output; max input; min input
function y = fcn(u,max,min)

y = (u - min)/(max - min);

== matlab function RealLifeTrainModel/CommSystem/SendMessageSystem/SendObs/Norm7 ==
  data: u input; y output; max input; min input
function y = fcn(u,max,min)

y = (u - min)/(max - min);

== matlab function RealLifeTrainModel/CommSystem/SendMessageSystem/SendObs/Norm8 ==
  data: u input; y output; max input; min input
function y = fcn(u,max,min)

y = (u - min)/(max - min);

== matlab function RealLifeTrainModel/CommSystem/SendMessageSystem/SendObs/Norm9 ==
  data: u input; y output; max input; min input
function y = fcn(u,max,min)

y = (u - min)/(max - min);

== matlab function RealLifeTrainModel/ContractionMetricFilterSystem2/Policy_SS/SmoothFnc1 ==
  data: u input; y output; smooth input
function y = fcn(u,smooth)
persistent last_value;

if(isempty(last_value))
    last_value = 0
end

y = smooth*last_value + (1 - smooth)*u
last_value = u

== matlab function RealLifeTrainModel/ContractionMetricFilterSystem2/Renormalize ==
  data: u input; y output
function y = fcn(u)

y = u*2 - 1;

== matlab function RealLifeTrainModel/MATLAB Function2 ==
  data: u input; y output; start input; time input
function y = fcn(u,start,time)

if((time - start) > 18)
    y=0
end
if((time - start) < 2)
    y = 0
else
    y = u

end

== matlab function RealLifeTrainModel/CommSystem/SendMessageSystem/SendObs1/CalcCrc ==
  data: u input; y output; length input
function y = fcn(u, length)
%#codegen

y = uint8(0);
length = length + 3;

for i = 1:length
    temp = (double(y) + double(u(i)))/2;  % safely add in double
    y = bitand(uint8(temp), uint8(255));  % clamp to 0-255, cast back to uint8
end

== matlab function RealLifeTrainModel/CommSystem/SendMessageSystem/SendObs1/Norm ==
  data: u input; y output; max input; min input
function y = fcn(u,max,min)

y = (u - min)/(max - min);

== matlab function RealLifeTrainModel/CommSystem/SendMessageSystem/SendObs1/Norm1 ==
  data: u input; y output; max input; min input
function y = fcn(u,max,min)

y = (u - min)/(max - min);

== matlab function RealLifeTrainModel/CommSystem/SendMessageSystem/SendObs1/Norm10 ==
  data: u input; y output; max input; min input
function y = fcn(u,max,min)

y = (u - min)/(max - min);

== matlab function RealLifeTrainModel/FunctionCalculateHydModel ==
  data: ixv input; f output; Pn input; Qn input; Un input; Vpl input; xp input; Pa input; Pb input; Ps input; Pt input; xpd input; g output; L_cyl input; Aa input; alfa input; c1 input; c2 input; Be input; flag_start input; d input; current input; dF_model output; cli input; g_med output; leak output

function [f,g,dF_model,g_med,leak] = fcn(ixv,Pn,Qn,Un,Vpl,xp,Pa,Pb,Ps,Pt,xpd,L_cyl,Aa,alfa,c1,c2,Be,flag_start,d,current,cli)

if flag_start == 1
    Kv = Qn/(Un*sqrt(Pn/2));
    
    Va = Vpl + Aa*xp;
    Vb = Vpl + (L_cyl - xp)*alfa*Aa;

    if(ixv >= 0)
        g = Be*Aa*Kv*( sign(Ps-Pa)*sqrt(abs(Ps-Pa))/Va + alfa*sign(Pb-Pt)*sqrt(abs(Pb-Pt))/Vb);
    else
        g = Be*Aa*Kv*( sign(Pa-Pt)*sqrt(abs(Pa-Pt))/Va + alfa*sign(Ps-Pb)*sqrt(abs(Ps-Pb))/Vb);
    end
    
    g1 = Be*Aa*Kv*( sign(Ps-Pa)*sqrt(abs(Ps-Pa))/Va + alfa*sign(Pb-Pt)*sqrt(abs(Pb-Pt))/Vb);
    g2 = Be*Aa*Kv*( sign(Pa-Pt)*sqrt(abs(Pa-Pt))/Va + alfa*sign(Ps-Pb)*sqrt(abs(Ps-Pb))/Vb);
    
    %g_med = (g1 + g2)/2;
    g_med = g;

    g_med = c2*g_med;

    f = -Be*Aa^2*(((alfa)^2)/Vb + 1/Va)*xpd;
    
    g = c2*g;
    f = c1*f;
    d = 0;
    leak = cli*(Pa - Pb)*Be*Aa*(1/Va + alfa/Vb);
    dF_model = f + g*current + g*d
else
    leak  =1;
    f = 1;
    g = 1;
    g_med = 1;
    dF_model = 0;
end

== matlab function RealLifeTrainModel/CommSystem/SendMessageSystem/SendObs1/Norm11 ==
  data: u input; y output; max input; min input
function y = fcn(u,max,min)

y = (u - min)/(max - min);

== matlab function RealLifeTrainModel/CommSystem/SendMessageSystem/SendObs1/Norm2 ==
  data: u input; y output; max input; min input
function y = fcn(u,max,min)

y = (u - min)/(max - min);

== matlab function RealLifeTrainModel/CommSystem/SendMessageSystem/SendObs1/Norm3 ==
  data: u input; y output; max input; min input
function y = fcn(u,max,min)

y = (u - min)/(max - min);

== matlab function RealLifeTrainModel/CommSystem/SendMessageSystem/SendObs1/Norm4 ==
  data: u input; y output; max input; min input
function y = fcn(u,max,min)

y = (u - min)/(max - min);

== matlab function RealLifeTrainModel/CommSystem/SendMessageSystem/SendObs1/Norm5 ==
  data: u input; y output; max input; min input
function y = fcn(u,max,min)

y = (u - min)/(max - min);

== matlab function RealLifeTrainModel/CommSystem/SendMessageSystem/SendObs1/Norm6 ==
  data: u input; y output; max input; min input
function y = fcn(u,max,min)

y = (u - min)/(max - min);

== matlab function RealLifeTrainModel/CommSystem/SendMessageSystem/SendObs1/Norm7 ==
  data: u input; y output; max input; min input
function y = fcn(u,max,min)

y = (u - min)/(max - min);

== matlab function RealLifeTrainModel/CommSystem/SendMessageSystem/SendObs1/Norm8 ==
  data: u input; y output; max input; min input
function y = fcn(u,max,min)

y = (u - min)/(max - min);

== matlab function RealLifeTrainModel/CommSystem/SendMessageSystem/SendObs1/Norm9 ==
  data: u input; y output; max input; min input
function y = fcn(u,max,min)

y = (u - min)/(max - min);
